simulink model "inpguitest"  (Simulink 8.6)
settings: Solver=FixedStepDiscrete  StartTime=0.0  StopTime=inf  RelTol=1e-3
settings Model: RequirementInfo="{}  %GIDa_a077a008_147d_4278_b137_64d319535cf1"  Creator=nskandan  LastModifiedBy=achal
settings OptimizationCC: ExpressionDepthLimit=128  InitFltsAndDblsToZero=on
settings DebuggingCC: SaveWithParameterizedLinksMsg=none  SignalResolutionControl=TryResolveAllWithWarning  FcnCallInpInsideContextMsg=UseLocalSettings  StateNameClashWarn=none  StrictBusMsg=Warning
settings GRTTargetCC: TargetFcnLib=ansi_tfl_tmw.mat  GeneratePreprocessorConditionals=Use local settings

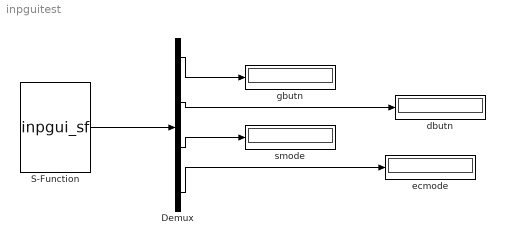
== system inpguitest ==
  Demux : Demux
  S-Function : S-Function  FunctionName=inpgui_sf  Parameters=0.005  SFunctionDeploymentMode=off  EnableBusSupport=off
  dbutn : Display
  ecmode : Display
  gbutn : Display
  smode : Display
  wires:
  S-Function/1 -> Demux/1
  Demux/1 -> gbutn/1
  Demux/2 -> dbutn/1
  Demux/3 -> smode/1
  Demux/4 -> ecmode/1
